simulink model "task_8"  (R2023a)
settings: Solver=VariableStepAuto  StartTime=0.0  StopTime=70  RelTol=1e-3  EnableMultiTasking=on
model workspace (MAT data in the model file):
  Tp = 1
  u_liner = 1
settings Model: Creator=Laptop  LastModifiedBy=denys
settings SolverCC: AlgebraicLoopSolver=TrustRegion
settings DataIOCC: ReturnWorkspaceOutputs=off
settings OptimizationCC: LifeSpan=inf
settings DebuggingCC: UnconnectedInputMsg=warning  UnconnectedOutputMsg=warning  UnconnectedLineMsg=warning  SFUnexpectedBacktrackingDiag=warning  SFNoUnconditionalDefaultTransitionDiag=warning  ArithmeticOperatorsInVariantConditions=warning
settings ModelReferenceCC: EnableRefExpFcnMdlSchedulingChecks=on
settings SFSimCC: SimUseLocalCustomCode=off  CustomCodeUndefinedFunction=UseInterfaceOnly
settings RTWCC: RTWUseLocalCustomCode=off
settings CodeAppCC: StateflowObjectComments=on
settings GRTTargetCC: TargetLangStandard=C89/C90 (ANSI)
settings ConfigComp: CovMetricSettings=dw  CovSaveCumulativeToWorkspaceVar=on  CovSaveSingleToWorkspaceVar=on  CovExternalEMLEnable=off

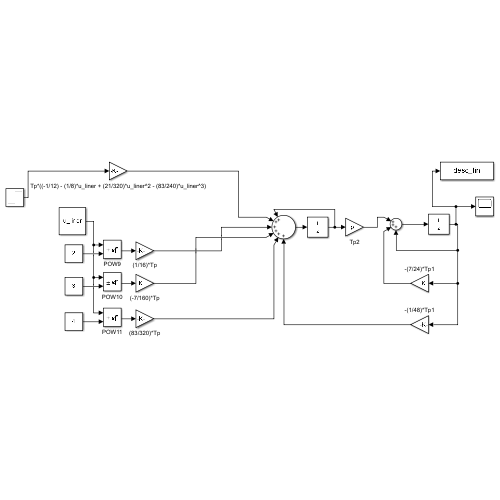
[thumbnail: Simulink's stored preview of the top-level diagram]
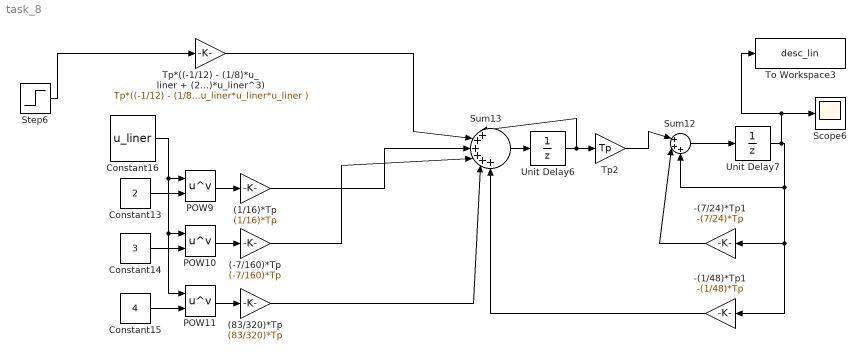
== system task_8 ==
  (-7/160)*Tp : Gain  Gain=(-7/160)*Tp
  (1/16)*Tp : Gain  Gain=(1/16)*Tp
  (83/320)*Tp : Gain  Gain=(83/320)*Tp
  -(1/48)*Tp1 : Gain  Gain=-(1/48)*Tp
  -(7/24)*Tp1 : Gain  Gain=-(7/24)*Tp
  Constant13 : Constant  Value=2
  Constant14 : Constant  Value=3
  Constant15 : Constant  Value=4
  Constant16 : Constant  Value=u_liner
  POW10 : Math  Operator=pow  SignedPower=on
  POW11 : Math  Operator=pow  SignedPower=on
  POW9 : Math  Operator=pow  SignedPower=on
  Scope6 : Scope
  Step6 : Step  After=3  SampleTime=Tp
  Sum12 : Sum  Inputs=|+++
  Sum13 : Sum  Inputs=|++++++
  To Workspace3 : ToWorkspace  VariableName=desc_lin  SaveFormat=Timeseries  SampleTime=-1
  Tp*((-1/12) - (1/8)*u_liner + (21/320)*u_liner^2 - (83/240)*u_liner^3) : Gain  Gain=Tp*((-1/12) - (1/8)*u_liner + (21/320)*u_liner*u_liner - (83/240)*u_liner*u_liner*u_liner )
  Tp2 : Gain  Gain=Tp
  Unit Delay6 : UnitDelay  SampleTime=Tp  HasFrameUpgradeWarning=on
  Unit Delay7 : UnitDelay  SampleTime=Tp  HasFrameUpgradeWarning=on
  wires:
  Constant13/1 -> POW9/2
  POW9/1 -> (1/16)*Tp/1
  Tp2/1 -> Sum12/1
  -(7/24)*Tp1/1 -> Sum12/2
  Sum12/1 -> Unit Delay7/1
  Constant15/1 -> POW11/2
  Unit Delay6/1 -> Sum13/1, Tp2/1
  POW10/1 -> (-7/160)*Tp/1
  Sum13/1 -> Unit Delay6/1
  Constant14/1 -> POW10/2
  Unit Delay7/1 -> To Workspace3/1, Scope6/1, -(1/48)*Tp1/1, -(7/24)*Tp1/1, Sum12/3
  Step6/1 -> Tp*((-1/12) - (1/8)*u_liner + (21/320)*u_liner^2 - (83/240)*u_liner^3)/1
  -(1/48)*Tp1/1 -> Sum13/6
  POW11/1 -> (83/320)*Tp/1
  Tp*((-1/12) - (1/8)*u_liner + (21/320)*u_liner^2 - (83/240)*u_liner^3)/1 -> Sum13/2
  (1/16)*Tp/1 -> Sum13/3
  (-7/160)*Tp/1 -> Sum13/4
  (83/320)*Tp/1 -> Sum13/5
  Constant16/1 -> POW11/1, POW10/1, POW9/1
